simulink model "Sim_Forcing_003h_expe_infra5_practice1"  (Simulink 7.4)
settings: Solver=FixedStepDiscrete  StartTime=0.0  StopTime=inf  FixedStep=0.004  RelTol=1e-3
undefined symbols (not defined in the file or in its folder): DiscIntNeverNeededParam
libraries: simulink x24, gt_rt_lib x20, xpcutilitieslib x3, xpclib x2
(part 2 of 3)

== system Sim_Forcing_003h_expe_infra5_practice1/BEC (May 7, 2015)/CAN Receive/Convert 4*uni8 to int3 ==
  byte0 : Inport
  byte1 : Inport  Port=2
  byte2 : Inport  Port=3
  byte3 : Inport  Port=4
  Add : Sum  Inputs=++++  OutDataTypeMode=int32  OutDataType=fixdt(1, 16)  OutScaling=2^-10  OutDataTypeStr=int32
  Gain2 : Gain  Gain=256  ParameterDataType=fixdt(1, 16)  ParameterScaling=2^0  OutDataType=fixdt(1, 16)  OutScaling=2^0
  Gain3 : Gain  Gain=2^16  ParameterDataType=fixdt(1, 16)  ParameterScaling=2^0  OutDataType=fixdt(1, 16)  OutScaling=2^0
  Gain4 : Gain  Gain=2^24  ParameterDataType=fixdt(1, 16)  ParameterScaling=2^0  OutDataType=fixdt(1, 16)  OutScaling=2^0
  int : Outport
  wires:
  Gain4/1 -> Add/4
  byte3/1 -> Gain4/1
  byte2/1 -> Gain3/1
  byte1/1 -> Gain2/1
  Add/1 -> int/1
  byte0/1 -> Add/1
  Gain3/1 -> Add/3
  Gain2/1 -> Add/2

== system Sim_Forcing_003h_expe_infra5_practice1/BEC (May 7, 2015)/CAN Receive/Convert 4*uni8 to int4 ==
  byte0 : Inport
  byte1 : Inport  Port=2
  byte2 : Inport  Port=3
  byte3 : Inport  Port=4
  Add : Sum  Inputs=++++  OutDataTypeMode=int32  OutDataType=fixdt(1, 16)  OutScaling=2^-10  OutDataTypeStr=int32
  Gain2 : Gain  Gain=256  ParameterDataType=fixdt(1, 16)  ParameterScaling=2^0  OutDataType=fixdt(1, 16)  OutScaling=2^0
  Gain3 : Gain  Gain=2^16  ParameterDataType=fixdt(1, 16)  ParameterScaling=2^0  OutDataType=fixdt(1, 16)  OutScaling=2^0
  Gain4 : Gain  Gain=2^24  ParameterDataType=fixdt(1, 16)  ParameterScaling=2^0  OutDataType=fixdt(1, 16)  OutScaling=2^0
  int : Outport
  wires:
  Gain2/1 -> Add/2
  Gain3/1 -> Add/3
  byte0/1 -> Add/1
  Add/1 -> int/1
  byte1/1 -> Gain2/1
  byte2/1 -> Gain3/1
  byte3/1 -> Gain4/1
  Gain4/1 -> Add/4

== system Sim_Forcing_003h_expe_infra5_practice1/BEC (May 7, 2015)/CAN Receive/Convert 4*uni8 to int5 ==
  byte0 : Inport
  byte1 : Inport  Port=2
  byte2 : Inport  Port=3
  byte3 : Inport  Port=4
  Add : Sum  Inputs=++++  OutDataTypeMode=int32  OutDataType=fixdt(1, 16)  OutScaling=2^-10  OutDataTypeStr=int32
  Gain2 : Gain  Gain=256  ParameterDataType=fixdt(1, 16)  ParameterScaling=2^0  OutDataType=fixdt(1, 16)  OutScaling=2^0
  Gain3 : Gain  Gain=2^16  ParameterDataType=fixdt(1, 16)  ParameterScaling=2^0  OutDataType=fixdt(1, 16)  OutScaling=2^0
  Gain4 : Gain  Gain=2^24  ParameterDataType=fixdt(1, 16)  ParameterScaling=2^0  OutDataType=fixdt(1, 16)  OutScaling=2^0
  int : Outport
  wires:
  Gain4/1 -> Add/4
  byte3/1 -> Gain4/1
  byte2/1 -> Gain3/1
  byte1/1 -> Gain2/1
  Add/1 -> int/1
  byte0/1 -> Add/1
  Gain3/1 -> Add/3
  Gain2/1 -> Add/2

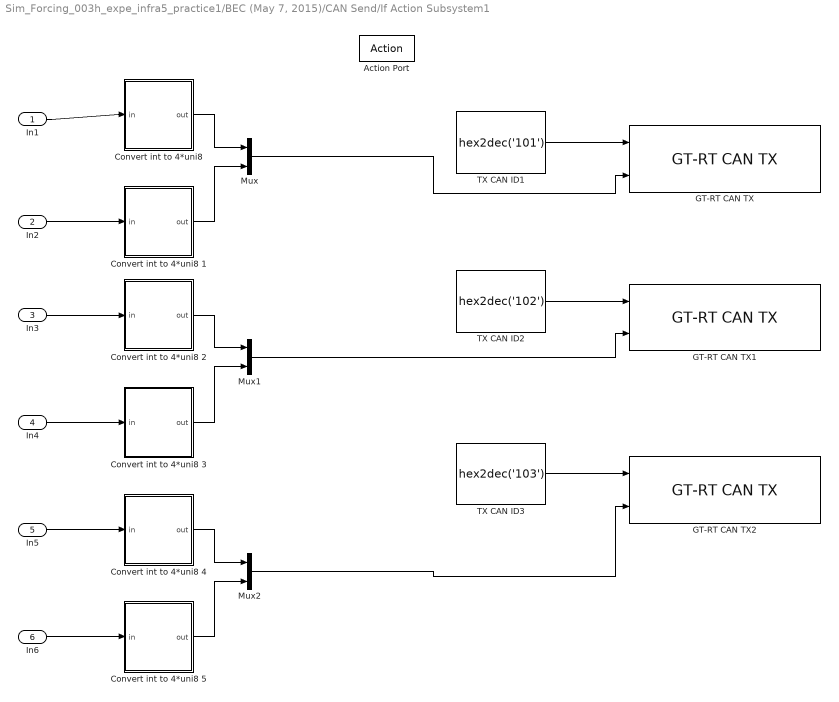
== system Sim_Forcing_003h_expe_infra5_practice1/BEC (May 7, 2015)/CAN Send/If Action Subsystem1 ==
  In1 : Inport  OutDataType=fixdt(1, 16)  OutScaling=2^0
  In2 : Inport  Port=2  OutDataType=fixdt(1, 16)  OutScaling=2^0
  In3 : Inport  Port=3  OutDataType=fixdt(1, 16)  OutScaling=2^0
  In4 : Inport  Port=4  OutDataType=fixdt(1, 16)  OutScaling=2^0
  In5 : Inport  Port=5  OutDataType=fixdt(1, 16)  OutScaling=2^0
  In6 : Inport  Port=6  OutDataType=fixdt(1, 16)  OutScaling=2^0
  Action Port : ActionPort  ActionType=then
  "Convert int to 4*uni8 " : Subsystem
  Convert int to 4*uni8 1 : Subsystem
  Convert int to 4*uni8 2 : Subsystem
  Convert int to 4*uni8 3 : Subsystem
  Convert int to 4*uni8 4 : Subsystem
  Convert int to 4*uni8 5 : Subsystem
  GT-RT CAN TX : gt_rt_lib/GT-RT CAN TX  uri='gt_rt_dev://localhost/dev/can0#0'  mff=MFF_11_DAT
  GT-RT CAN TX1 : gt_rt_lib/GT-RT CAN TX  uri='gt_rt_dev://localhost/dev/can0#0'  mff=MFF_11_DAT
  GT-RT CAN TX2 : gt_rt_lib/GT-RT CAN TX  uri='gt_rt_dev://localhost/dev/can0#0'  mff=MFF_11_DAT
  Mux : Mux  Inputs=2
  Mux1 : Mux  Inputs=2
  Mux2 : Mux  Inputs=2
  TX CAN ID1 : Constant  Value=hex2dec('101')  OutDataTypeMode=uint32  OutDataType=sfix(16)  OutScaling=2^0  OutDataTypeStr=uint32
  TX CAN ID2 : Constant  Value=hex2dec('102')  OutDataTypeMode=uint32  OutDataType=sfix(16)  OutScaling=2^0  OutDataTypeStr=uint32
  TX CAN ID3 : Constant  Value=hex2dec('103')  OutDataTypeMode=uint32  OutDataType=sfix(16)  OutScaling=2^0  OutDataTypeStr=uint32
  wires:
  In1/1 -> "Convert int to 4*uni8 "/1(in)
  In2/1 -> Convert int to 4*uni8 1/1(in)
  In3/1 -> Convert int to 4*uni8 2/1(in)
  In4/1 -> Convert int to 4*uni8 3/1(in)
  In5/1 -> Convert int to 4*uni8 4/1(in)
  In6/1 -> Convert int to 4*uni8 5/1(in)
  Mux2/1 -> GT-RT CAN TX2/2
  Convert int to 4*uni8 5/1(out) -> Mux2/2
  Convert int to 4*uni8 4/1(out) -> Mux2/1
  Mux1/1 -> GT-RT CAN TX1/2
  Convert int to 4*uni8 3/1(out) -> Mux1/2
  Convert int to 4*uni8 2/1(out) -> Mux1/1
  Mux/1 -> GT-RT CAN TX/2
  Convert int to 4*uni8 1/1(out) -> Mux/2
  "Convert int to 4*uni8 "/1(out) -> Mux/1
  TX CAN ID3/1 -> GT-RT CAN TX2/1
  TX CAN ID2/1 -> GT-RT CAN TX1/1
  TX CAN ID1/1 -> GT-RT CAN TX/1

== system Sim_Forcing_003h_expe_infra5_practice1/BEC (May 7, 2015)/Software limit switches/Subsystem ==
  In1 : Inport
  act : Inport  Port=2
  Abs1 : Abs  OutDataType=fixdt(1, 16)  OutScaling=2^0
  Abs2 : Abs  OutDataType=fixdt(1, 16)  OutScaling=2^0
  Add1 : Sum  Inputs=+-  OutDataType=fixdt(1, 16)  OutScaling=2^-10
  Add2 : Sum  Inputs=-+  OutDataType=fixdt(1, 16)  OutScaling=2^-10
  Display : Display
  Display2 : Display
  If Action Subsystem : Subsystem  TreatAsAtomicUnit=on
  If Action Subsystem1 : Subsystem  TreatAsAtomicUnit=on
  If2 : If
  NSEA1 : Constant  Value=-160  OutDataType=fixdt(1, 16)  OutScaling=2^0
  PSEA1 : Constant  Value=160  OutDataType=fixdt(1, 16)  OutScaling=2^0
  Switch : Switch  Criteria=u2 > Threshold  OutDataType=fixdt(1, 16)  OutScaling=2^0
  Switch1 : Switch  Criteria=u2 ~= 0  OutDataType=fixdt(1, 16)  OutScaling=2^0
  Out1 : Outport
  wires:
  If Action Subsystem1/1(Out1) -> Switch/3
  If Action Subsystem/1(Out1) -> Display/1, Switch/1
  Abs1/1 -> If Action Subsystem1/2(dif)
  If2/2 -> If Action Subsystem1/Action
  If2/1 -> If Action Subsystem/Action
  In1/1 -> If2/1, If Action Subsystem/2(Inc), If Action Subsystem1/1(Inc), Switch/2, Switch1/2, Switch1/3
  Abs2/1 -> If Action Subsystem/1(dif)
  NSEA1/1 -> Add1/2
  PSEA1/1 -> Add2/1
  Add1/1 -> Abs1/1
  Add2/1 -> Abs2/1
  Switch/1 -> Switch1/1
  Switch1/1 -> Out1/1, Display2/1
  act/1 -> Add1/1, Add2/2

== system Sim_Forcing_003h_expe_infra5_practice1/BEC (May 7, 2015)/Software limit switches/Subsystem1 ==
  In1 : Inport
  act : Inport  Port=2
  Abs1 : Abs  OutDataType=fixdt(1, 16)  OutScaling=2^0
  Abs2 : Abs  OutDataType=fixdt(1, 16)  OutScaling=2^0
  Add1 : Sum  Inputs=+-  OutDataType=fixdt(1, 16)  OutScaling=2^-10
  Add2 : Sum  Inputs=-+  OutDataType=fixdt(1, 16)  OutScaling=2^-10
  If Action Subsystem : Subsystem  TreatAsAtomicUnit=on
  If Action Subsystem1 : Subsystem  TreatAsAtomicUnit=on
  If2 : If
  NSEA1 : Constant  Value=-130  OutDataType=fixdt(1, 16)  OutScaling=2^0
  PSEA1 : Constant  Value=20  OutDataType=fixdt(1, 16)  OutScaling=2^0
  Switch : Switch  OutDataType=fixdt(1, 16)  OutScaling=2^0
  Switch1 : Switch  Criteria=u2 ~= 0  OutDataType=fixdt(1, 16)  OutScaling=2^0
  Out1 : Outport
  wires:
  act/1 -> Add1/1, Add2/2
  Add2/1 -> Abs2/1
  Add1/1 -> Abs1/1
  PSEA1/1 -> Add2/1
  NSEA1/1 -> Add1/2
  Abs2/1 -> If Action Subsystem/1(dif)
  In1/1 -> If Action Subsystem1/1(Inc), If Action Subsystem/2(Inc), Switch/2, Switch1/2, Switch1/3, If2/1
  If2/1 -> If Action Subsystem/Action
  If2/2 -> If Action Subsystem1/Action
  Abs1/1 -> If Action Subsystem1/2(dif)
  If Action Subsystem/1(Out1) -> Switch/1
  If Action Subsystem1/1(Out1) -> Switch/3
  Switch/1 -> Switch1/1
  Switch1/1 -> Out1/1

== system Sim_Forcing_003h_expe_infra5_practice1/BEC (May 7, 2015)/Software limit switches/Subsystem2 ==
  In1 : Inport
  act : Inport  Port=2
  Abs1 : Abs  OutDataType=fixdt(1, 16)  OutScaling=2^0
  Abs2 : Abs  OutDataType=fixdt(1, 16)  OutScaling=2^0
  Add1 : Sum  Inputs=+-  OutDataType=fixdt(1, 16)  OutScaling=2^-10
  Add2 : Sum  Inputs=-+  OutDataType=fixdt(1, 16)  OutScaling=2^-10
  If Action Subsystem : Subsystem  TreatAsAtomicUnit=on
  If Action Subsystem1 : Subsystem  TreatAsAtomicUnit=on
  If2 : If
  NSEA1 : Constant  Value=-88  OutDataType=fixdt(1, 16)  OutScaling=2^0
  PSEA1 : Constant  Value=88  OutDataType=fixdt(1, 16)  OutScaling=2^0
  Switch : Switch  OutDataType=fixdt(1, 16)  OutScaling=2^0
  Switch1 : Switch  Criteria=u2 ~= 0  OutDataType=fixdt(1, 16)  OutScaling=2^0
  Out1 : Outport
  wires:
  If Action Subsystem1/1(Out1) -> Switch/3
  If Action Subsystem/1(Out1) -> Switch/1
  Abs1/1 -> If Action Subsystem1/2(dif)
  If2/2 -> If Action Subsystem1/Action
  If2/1 -> If Action Subsystem/Action
  In1/1 -> If2/1, If Action Subsystem/2(Inc), If Action Subsystem1/1(Inc), Switch/2, Switch1/2, Switch1/3
  Abs2/1 -> If Action Subsystem/1(dif)
  NSEA1/1 -> Add1/2
  PSEA1/1 -> Add2/1
  Add1/1 -> Abs1/1
  Add2/1 -> Abs2/1
  act/1 -> Add1/1, Add2/2
  Switch/1 -> Switch1/1
  Switch1/1 -> Out1/1

== system Sim_Forcing_003h_expe_infra5_practice1/BEC (May 7, 2015)/Software limit switches/Subsystem3 ==
  In1 : Inport
  act : Inport  Port=2
  Abs1 : Abs  OutDataType=fixdt(1, 16)  OutScaling=2^0
  Abs2 : Abs  OutDataType=fixdt(1, 16)  OutScaling=2^0
  Add1 : Sum  Inputs=+-  OutDataType=fixdt(1, 16)  OutScaling=2^-10
  Add2 : Sum  Inputs=-+  OutDataType=fixdt(1, 16)  OutScaling=2^-10
  If Action Subsystem : Subsystem  TreatAsAtomicUnit=on
  If Action Subsystem1 : Subsystem  TreatAsAtomicUnit=on
  If2 : If
  NSEA1 : Constant  Value=-350  OutDataType=fixdt(1, 16)  OutScaling=2^0
  PSEA1 : Constant  Value=350  OutDataType=fixdt(1, 16)  OutScaling=2^0
  Switch : Switch  OutDataType=fixdt(1, 16)  OutScaling=2^0
  Switch1 : Switch  Criteria=u2 ~= 0  OutDataType=fixdt(1, 16)  OutScaling=2^0
  Out1 : Outport
  wires:
  Add2/1 -> Abs2/1
  Add1/1 -> Abs1/1
  PSEA1/1 -> Add2/1
  NSEA1/1 -> Add1/2
  Abs2/1 -> If Action Subsystem/1(dif)
  In1/1 -> If Action Subsystem1/1(Inc), If Action Subsystem/2(Inc), Switch/2, Switch1/2, Switch1/3, If2/1
  If2/1 -> If Action Subsystem/Action
  If2/2 -> If Action Subsystem1/Action
  act/1 -> Add2/2, Add1/1
  Abs1/1 -> If Action Subsystem1/2(dif)
  If Action Subsystem/1(Out1) -> Switch/1
  If Action Subsystem1/1(Out1) -> Switch/3
  Switch/1 -> Switch1/1
  Switch1/1 -> Out1/1

== system Sim_Forcing_003h_expe_infra5_practice1/BEC (May 7, 2015)/Software limit switches/Subsystem4 ==
  In1 : Inport
  act : Inport  Port=2
  Abs1 : Abs  OutDataType=fixdt(1, 16)  OutScaling=2^0
  Abs2 : Abs  OutDataType=fixdt(1, 16)  OutScaling=2^0
  Add1 : Sum  Inputs=+-  OutDataType=fixdt(1, 16)  OutScaling=2^-10
  Add2 : Sum  Inputs=-+  OutDataType=fixdt(1, 16)  OutScaling=2^-10
  If Action Subsystem : Subsystem  TreatAsAtomicUnit=on
  If Action Subsystem1 : Subsystem  TreatAsAtomicUnit=on
  If2 : If
  NSEA1 : Constant  Value=-61  OutDataType=fixdt(1, 16)  OutScaling=2^0
  PSEA1 : Constant  Value=61  OutDataType=fixdt(1, 16)  OutScaling=2^0
  Switch : Switch  OutDataType=fixdt(1, 16)  OutScaling=2^0
  Switch1 : Switch  Criteria=u2 ~= 0  OutDataType=fixdt(1, 16)  OutScaling=2^0
  Out1 : Outport
  wires:
  If Action Subsystem/1(Out1) -> Switch/1
  Abs1/1 -> If Action Subsystem1/2(dif)
  If2/2 -> If Action Subsystem1/Action
  If2/1 -> If Action Subsystem/Action
  In1/1 -> If2/1, If Action Subsystem/2(Inc), If Action Subsystem1/1(Inc), Switch/2, Switch1/2, Switch1/3
  Abs2/1 -> If Action Subsystem/1(dif)
  NSEA1/1 -> Add1/2
  PSEA1/1 -> Add2/1
  Add1/1 -> Abs1/1
  Add2/1 -> Abs2/1
  If Action Subsystem1/1(Out1) -> Switch/3
  Switch/1 -> Switch1/1
  Switch1/1 -> Out1/1
  act/1 -> Add2/2, Add1/1

== system Sim_Forcing_003h_expe_infra5_practice1/BEC (May 7, 2015)/Software limit switches/Subsystem5 ==
  In1 : Inport
  act : Inport  Port=2
  Abs1 : Abs  OutDataType=fixdt(1, 16)  OutScaling=2^0
  Abs2 : Abs  OutDataType=fixdt(1, 16)  OutScaling=2^0
  Add1 : Sum  Inputs=+-  OutDataType=fixdt(1, 16)  OutScaling=2^-10
  Add2 : Sum  Inputs=-+  OutDataType=fixdt(1, 16)  OutScaling=2^-10
  If Action Subsystem : Subsystem  TreatAsAtomicUnit=on
  If Action Subsystem1 : Subsystem  TreatAsAtomicUnit=on
  If2 : If
  NSEA1 : Constant  Value=-350  OutDataType=fixdt(1, 16)  OutScaling=2^0
  PSEA1 : Constant  Value=350  OutDataType=fixdt(1, 16)  OutScaling=2^0
  Switch : Switch  OutDataType=fixdt(1, 16)  OutScaling=2^0
  Switch1 : Switch  Criteria=u2 ~= 0  OutDataType=fixdt(1, 16)  OutScaling=2^0
  Out1 : Outport
  wires:
  Add2/1 -> Abs2/1
  Add1/1 -> Abs1/1
  PSEA1/1 -> Add2/1
  NSEA1/1 -> Add1/2
  Abs2/1 -> If Action Subsystem/1(dif)
  In1/1 -> If Action Subsystem1/1(Inc), If Action Subsystem/2(Inc), Switch/2, Switch1/2, Switch1/3, If2/1
  If2/1 -> If Action Subsystem/Action
  If2/2 -> If Action Subsystem1/Action
  Abs1/1 -> If Action Subsystem1/2(dif)
  If Action Subsystem/1(Out1) -> Switch/1
  If Action Subsystem1/1(Out1) -> Switch/3
  Switch/1 -> Switch1/1
  Switch1/1 -> Out1/1
  act/1 -> Add2/2, Add1/1

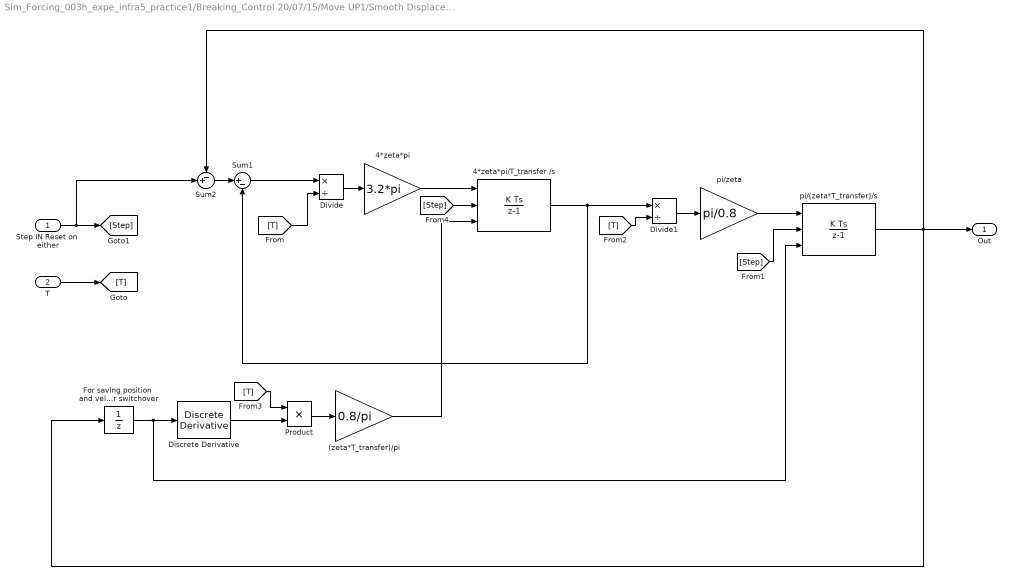
== system Sim_Forcing_003h_expe_infra5_practice1/Breaking_Control 20/07/15/Move UP1/Smooth Displacement Second-Order Filter, zeta 0.8 ==
  Step IN Reset on  either : Inport
  T : Inport  Port=2  OutDataType=fixdt(1, 16)  OutScaling=2^0
  (zeta*T_transfer)/pi : Gain  Gain=0.8/pi  ParameterDataType=fixdt(1, 16)  ParameterScaling=2^0  OutDataType=fixdt(1, 16)  OutScaling=2^0
  4*zeta*pi : Gain  Gain=3.2*pi  ParameterDataType=fixdt(1, 16)  ParameterScaling=2^0  OutDataType=fixdt(1, 16)  OutScaling=2^0
  4*zeta*pi/T_transfer /s : DiscreteIntegrator  gainval=1  ExternalReset=either  InitialConditionSource=external  SampleTime=0.004  OutDataType=fixdt(1, 16)  OutScaling=2^0  ICPrevOutput=DiscIntNeverNeededParam  ICPrevScaledInput=DiscIntNeverNeededParam
  Discrete Derivative : simulink/Discrete/Discrete Derivative  SystemSampleTime=-1  gainval=1.0  ICPrevScaledInput=0.0  OutMin=[]  OutMax=[]  OutDataType=fixdt(1, 16)  OutScaling=2^-10  DoSatur=off
  Divide : Product  Inputs=*/  OutDataType=fixdt(1, 16)  OutScaling=2^-10
  Divide1 : Product  Inputs=*/  OutDataType=fixdt(1, 16)  OutScaling=2^-10
  For saving position  and velocity until after switchover : UnitDelay  SampleTime=-1
  Product : Product  OutDataType=fixdt(1, 16)  OutScaling=2^0  RndMeth=Zero
  Sum1 : Sum  Inputs=|+-  OutDataType=fixdt(1, 16)  OutScaling=2^0
  Sum2 : Sum  Inputs=-+|  OutDataType=fixdt(1, 16)  OutScaling=2^0
  pi/(zeta*T_transfer)/s : DiscreteIntegrator  gainval=1  ExternalReset=either  InitialConditionSource=external  SampleTime=0.004  OutDataType=fixdt(1, 16)  OutScaling=2^0  ICPrevOutput=DiscIntNeverNeededParam  ICPrevScaledInput=DiscIntNeverNeededParam
  pi/zeta : Gain  Gain=pi/0.8  ParameterDataType=fixdt(1, 16)  ParameterScaling=2^0  OutDataType=fixdt(1, 16)  OutScaling=2^0
  Out : Outport
  wires:
  Discrete Derivative/1 -> Product/2
  Product/1 -> (zeta*T_transfer)/pi/1
  Divide/1 -> 4*zeta*pi/1
  Divide1/1 -> pi/zeta/1
  pi/zeta/1 -> pi/(zeta*T_transfer)/s/1
  pi/(zeta*T_transfer)/s/1 -> Sum2/1, Out/1, For saving position  and velocity until after switchover/1
  4*zeta*pi/T_transfer /s/1 -> Divide1/1, Sum1/2
  Sum1/1 -> Divide/1
  4*zeta*pi/1 -> 4*zeta*pi/T_transfer /s/1
  T/1 -> [T]
  Step IN Reset on  either/1 -> [Step], Sum2/2
  [Step] -> 4*zeta*pi/T_transfer /s/2
  [Step] -> pi/(zeta*T_transfer)/s/2
  [T] -> Divide/2
  For saving position  and velocity until after switchover/1 -> Discrete Derivative/1, pi/(zeta*T_transfer)/s/3
  [T] -> Product/1
  (zeta*T_transfer)/pi/1 -> 4*zeta*pi/T_transfer /s/3
  [T] -> Divide1/2
  Sum2/1 -> Sum1/1

== system Sim_Forcing_003h_expe_infra5_practice1/Breaking_Control 20/07/15/Move UP1/add x_offset ==
  x_offset : Inport
  set_in : Inport  Port=2
  Embedded MATLAB Function : Stateflow chart
  set_out : Outport
  wires:
  x_offset/1 -> Embedded MATLAB Function/1(dx)
  Embedded MATLAB Function/1(set_out) -> set_out/1
  set_in/1 -> Embedded MATLAB Function/2(set_in)

== system Sim_Forcing_003h_expe_infra5_practice1/Breaking_Control 20/07/15/practice_phase1/Rate Control Dynamics Phi ==
  Turn_rate_roll (deg/sec) : Inport
  practice : Inport  Port=2
  reset from_connect_y : Inport  Port=3
  Constant : Constant  Value=0.1  OutDataType=fixdt(1, 16)  OutScaling=2^0
  Constant1 : Constant  Value=15  OutDataType=fixdt(1, 16)  OutScaling=2^0
  Constant3 : Constant  Value=0.1  OutDataType=fixdt(1, 16)  OutScaling=2^0
  Discrete-Time Integrator1 : DiscreteIntegrator  ExternalReset=either  SampleTime=0.004  OutDataType=fixdt(1, 16)  OutScaling=2^0  ICPrevOutput=DiscIntNeverNeededParam  ICPrevScaledInput=DiscIntNeverNeededParam
  Limit to 5 : Saturate  UpperLimit=5  LowerLimit=-5  OutDataType=fixdt(1, 16)  OutScaling=2^0
  Product : Product  OutDataType=fixdt(1, 16)  OutScaling=2^0  RndMeth=Zero
  "Second-Order Filter, zeta 0.8" : Subsystem
  "Smooth Displacement Second-Order Filter, zeta 0.8" : Subsystem
  Switch : Switch  Criteria=u2 > Threshold  OutDataType=fixdt(1, 16)  OutScaling=2^0
  phi (deg) : Outport
  wires:
  Turn_rate_roll (deg/sec)/1 -> "Second-Order Filter, zeta 0.8"/1(u)
  "Second-Order Filter, zeta 0.8"/1(x) -> Limit to 5/1
  Constant/1 -> "Second-Order Filter, zeta 0.8"/2(T)
  Discrete-Time Integrator1/1 -> Product/1
  Product/1 -> phi (deg)/1
  "Smooth Displacement Second-Order Filter, zeta 0.8"/1(Out) -> Product/2
  Limit to 5/1 -> Discrete-Time Integrator1/1
  practice/1 -> "Smooth Displacement Second-Order Filter, zeta 0.8"/1(Step IN Reset on  either), Switch/2
  reset from_connect_y/1 -> Discrete-Time Integrator1/2
  Constant3/1 -> Switch/1
  Constant1/1 -> Switch/3
  Switch/1 -> "Smooth Displacement Second-Order Filter, zeta 0.8"/2(T)

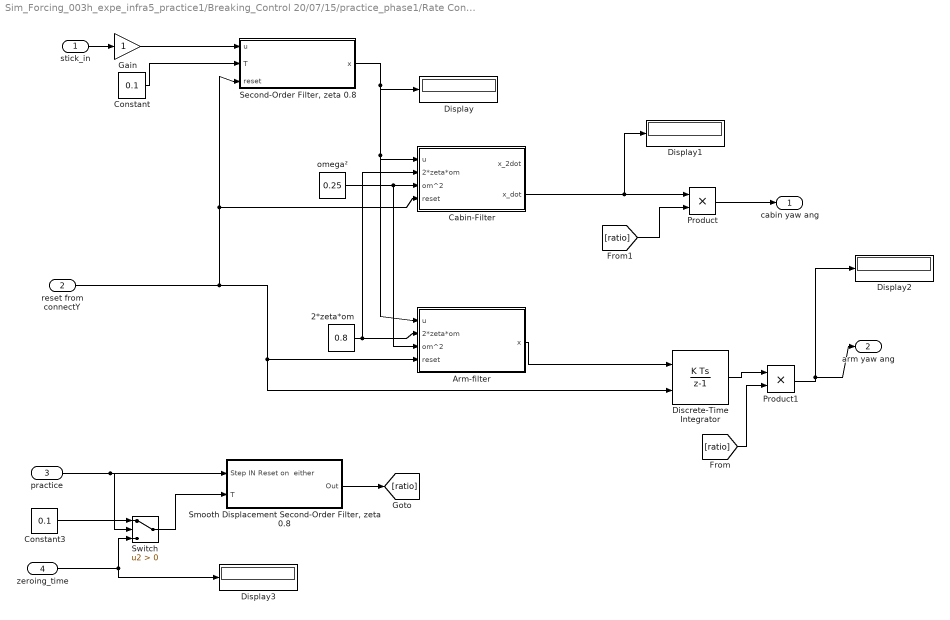
== system Sim_Forcing_003h_expe_infra5_practice1/Breaking_Control 20/07/15/practice_phase1/Rate Control Dynamics Psi2 ==
  stick_in : Inport  OutDataType=fixdt(1, 16)  OutScaling=2^0
  reset from connectY : Inport  Port=2  OutDataType=fixdt(1, 16)  OutScaling=2^0
  practice : Inport  Port=3
  zeroing_time : Inport  Port=4
  2*zeta*om : Constant  Value=0.8
  Arm-filter : Subsystem
  Cabin-Filter : Subsystem
  Constant : Constant  Value=0.1  OutDataType=fixdt(1, 16)  OutScaling=2^0
  Constant3 : Constant  Value=0.1  OutDataType=fixdt(1, 16)  OutScaling=2^0
  Discrete-Time Integrator : DiscreteIntegrator  ExternalReset=either  SampleTime=0.004  ICPrevOutput=DiscIntNeverNeededParam  ICPrevScaledInput=DiscIntNeverNeededParam
  Display{,1..3} (4 alike) : Display
  Gain : Gain  ParameterDataType=fixdt(1, 16)  ParameterScaling=2^0  OutDataType=fixdt(1, 16)  OutScaling=2^0
  Product : Product  OutDataType=fixdt(1, 16)  OutScaling=2^0  RndMeth=Zero
  Product1 : Product  OutDataType=fixdt(1, 16)  OutScaling=2^0  RndMeth=Zero
  "Second-Order Filter, zeta 0.8" : Subsystem
  "Smooth Displacement Second-Order Filter, zeta 0.8" : Subsystem
  Switch : Switch  Criteria=u2 > Threshold  OutDataType=fixdt(1, 16)  OutScaling=2^0
  omega² : Constant  Value=0.25
  cabin yaw ang : Outport  OutDataType=fixdt(1, 16)  OutScaling=2^0
  arm yaw ang : Outport  Port=2  OutDataType=fixdt(1, 16)  OutScaling=2^0
  wires:
  Arm-filter/1(x) -> Discrete-Time Integrator/1
  stick_in/1 -> Gain/1
  omega²/1 -> Arm-filter/3(om^2), Cabin-Filter/3(om^2)
  2*zeta*om/1 -> Arm-filter/2(2*zeta*om), Cabin-Filter/2(2*zeta*om)
  Cabin-Filter/2(x_dot) -> Display1/1, Product/1
  reset from connectY/1 -> Cabin-Filter/4(reset), "Second-Order Filter, zeta 0.8"/3(reset), Arm-filter/4(reset), Discrete-Time Integrator/2
  Constant/1 -> "Second-Order Filter, zeta 0.8"/2(T)
  "Second-Order Filter, zeta 0.8"/1(x) -> Cabin-Filter/1(u), Arm-filter/1(u), Display/1
  Gain/1 -> "Second-Order Filter, zeta 0.8"/1(u)
  Constant3/1 -> Switch/1
  zeroing_time/1 -> Switch/3, Display3/1
  Switch/1 -> "Smooth Displacement Second-Order Filter, zeta 0.8"/2(T)
  practice/1 -> Switch/2, "Smooth Displacement Second-Order Filter, zeta 0.8"/1(Step IN Reset on  either)
  "Smooth Displacement Second-Order Filter, zeta 0.8"/1(Out) -> [ratio]
  Product/1 -> cabin yaw ang/1
  Discrete-Time Integrator/1 -> Product1/1
  Product1/1 -> Display2/1, arm yaw ang/1
  [ratio] -> Product1/2
  [ratio] -> Product/2

== system Sim_Forcing_003h_expe_infra5_practice1/Breaking_Control 20/07/15/practice_phase1/Rate Control Dynamics Theta ==
  Turn_rate_pitch (deg/sec) : Inport
  practice : Inport  Port=2
  reset from_connect_y : Inport  Port=3
  Constant : Constant  Value=0.1  OutDataType=fixdt(1, 16)  OutScaling=2^0
  Constant1 : Constant  Value=15  OutDataType=fixdt(1, 16)  OutScaling=2^0
  Constant2 : Constant  Value=0.1  OutDataType=fixdt(1, 16)  OutScaling=2^0
  Discrete-Time Integrator1 : DiscreteIntegrator  ExternalReset=either  SampleTime=0.004  OutDataType=fixdt(1, 16)  OutScaling=2^0  ICPrevOutput=DiscIntNeverNeededParam  ICPrevScaledInput=DiscIntNeverNeededParam
  Limit to 5 : Saturate  UpperLimit=5  LowerLimit=-5  OutDataType=fixdt(1, 16)  OutScaling=2^0
  Product : Product  OutDataType=fixdt(1, 16)  OutScaling=2^0  RndMeth=Zero
  "Second-Order Filter, zeta 0.8" : Subsystem
  "Smooth Displacement Second-Order Filter, zeta 0.8" : Subsystem
  Switch : Switch  Criteria=u2 > Threshold  OutDataType=fixdt(1, 16)  OutScaling=2^0
  theta (deg) : Outport
  wires:
  Turn_rate_pitch (deg/sec)/1 -> "Second-Order Filter, zeta 0.8"/1(u)
  "Second-Order Filter, zeta 0.8"/1(x) -> Limit to 5/1
  Constant/1 -> "Second-Order Filter, zeta 0.8"/2(T)
  Discrete-Time Integrator1/1 -> Product/1
  Product/1 -> theta (deg)/1
  "Smooth Displacement Second-Order Filter, zeta 0.8"/1(Out) -> Product/2
  Limit to 5/1 -> Discrete-Time Integrator1/1
  reset from_connect_y/1 -> Discrete-Time Integrator1/2
  practice/1 -> "Smooth Displacement Second-Order Filter, zeta 0.8"/1(Step IN Reset on  either), Switch/2
  Switch/1 -> "Smooth Displacement Second-Order Filter, zeta 0.8"/2(T)
  Constant2/1 -> Switch/1
  Constant1/1 -> Switch/3

== system Sim_Forcing_003h_expe_infra5_practice1/Joint Controller (May 7, 2015)1/Forward Kinematics/KUKA2NED ==
  KUKA : Inport
  Constant : Constant  Value=[0 0 0 0 0 15.89]  OutDataType=fixdt(1, 16)  OutScaling=2^0
  Gain : Gain  Gain=[1 -1 -1 -1 -1 -1]  ParameterDataType=fixdt(1, 16)  ParameterScaling=2^0  OutDataType=fixdt(1, 16)  OutScaling=2^0
  Sum : Sum  Inputs=|++  OutDataType=fixdt(1, 16)  OutScaling=2^0
  NED : Outport
  wires:
  Gain/1 -> Sum/1
  KUKA/1 -> Gain/1
  Sum/1 -> NED/1
  Constant/1 -> Sum/2

== system Sim_Forcing_003h_expe_infra5_practice1/Joint Controller (May 7, 2015)1/Inverse Kinematics May 6, 2015/Inverse Kinematics ==
  note: (6_DOF_ACT - 6_DOF_COM) exp(-0.1t) + 6_DOF_COM
  vec : Inport
  Activate full inverse : Inport  Port=2
  6_DOF_ACT : Inport  Port=3  OutDataType=fixdt(1, 16)  OutScaling=2^0
  Demux : Demux  Outputs=[6,6]
  Discrete-Time Integrator : DiscreteIntegrator  gainval=1  ExternalReset=either  InitialConditionSource=external  SampleTime=-1  OutDataType=fixdt(1, 16)  OutScaling=2^0  ICPrevOutput=DiscIntNeverNeededParam  ICPrevScaledInput=DiscIntNeverNeededParam
  Gain : Gain  Gain=-0.1  ParameterDataType=fixdt(1, 16)  ParameterScaling=2^0  OutDataType=fixdt(1, 16)  OutScaling=2^0
  Mux : Mux  Inputs=2
  Select -6_DOF_COM : Selector  InputPortWidth=12  IndexOptions=Index vector (dialog)  Indices=[1 2 3 4 5 6]  OutputSizes=1
  Sum : Sum  Inputs=|-+  OutDataType=fixdt(1, 16)  OutScaling=2^0
  Sum1 : Sum  Inputs=|++  OutDataType=fixdt(1, 16)  OutScaling=2^0
  full inverse kin : Subsystem
  out : Outport  OutDataType=fixdt(1, 16)  OutScaling=2^0
  wires:
  vec/1 -> Select -6_DOF_COM/1, Demux/1
  full inverse kin/1(out) -> out/1
  Activate full inverse/1 -> full inverse kin/Enable, Discrete-Time Integrator/2
  Discrete-Time Integrator/1 -> Gain/1, Sum1/2
  Gain/1 -> Discrete-Time Integrator/1
  6_DOF_ACT/1 -> Sum/2
  Select -6_DOF_COM/1 -> Sum/1
  Sum/1 -> Discrete-Time Integrator/3
  Demux/2 -> Mux/2
  Demux/1 -> Sum1/1
  Sum1/1 -> Mux/1
  Mux/1 -> full inverse kin/1(vec)

== system Sim_Forcing_003h_expe_infra5_practice1/Joint Controller (May 7, 2015)1/Inverse Kinematics May 6, 2015/NED2KUKA ==
  NED : Inport
  Constant : Constant  Value=[0 0 0 0 0 15.89]  OutDataType=fixdt(1, 16)  OutScaling=2^0
  Gain : Gain  Gain=[1 -1 -1 -1 -1 -1]  ParameterDataType=fixdt(1, 16)  ParameterScaling=2^0  OutDataType=fixdt(1, 16)  OutScaling=2^0
  Sum : Sum  Inputs=|++  OutDataType=fixdt(1, 16)  OutScaling=2^0
  KUKA : Outport
  wires:
  Gain/1 -> Sum/1
  NED/1 -> Gain/1
  Sum/1 -> KUKA/1
  Constant/1 -> Sum/2

== system Sim_Forcing_003h_expe_infra5_practice1/Joint Controller (May 7, 2015)1/Inverse Kinematics May 6, 2015/Simplified Inverse Kinematics ==
  note: (A1-A6_ACT - A1-A6_COM) exp(-0.1t) + A1-A6_COM
  note: Selects and sets
      |  A1, A4,A6 to zero
  note: This version has been tested on May 6, 2015
  activate simplified : Inport  OutDataType=fixdt(1, 16)  OutScaling=2^0
  vec : Inport  Port=2  OutDataType=fixdt(1, 16)  OutScaling=2^0
  A1-A6 ACT : Selector  InputPortWidth=12  IndexOptions=Index vector (dialog)  Indices=[7 8 9 10 11 12]  OutputSizes=1
  A1-A6 COM : Subsystem
  Discrete-Time Integrator1 : DiscreteIntegrator  gainval=1  ExternalReset=either  InitialConditionSource=external  SampleTime=-1  OutDataType=fixdt(1, 16)  OutScaling=2^0  ICPrevOutput=DiscIntNeverNeededParam  ICPrevScaledInput=DiscIntNeverNeededParam
  Gain1 : Gain  Gain=-0.1  ParameterDataType=fixdt(1, 16)  ParameterScaling=2^0  OutDataType=fixdt(1, 16)  OutScaling=2^0
  Mux : Mux  Inputs=2
  N : Selector  InputPortWidth=7  IndexOptions=Index vector (dialog)  Indices=7  OutputSizes=1
  Simplified Inverse Kin : Subsystem
  Sum : Sum  Inputs=-+|  OutDataType=fixdt(1, 16)  OutScaling=2^0
  Sum1 : Sum  Inputs=++|  OutDataType=fixdt(1, 16)  OutScaling=2^0
  out : Outport  OutDataType=fixdt(1, 16)  OutScaling=2^0
  wires:
  vec/1 -> Simplified Inverse Kin/1(Vec), A1-A6 ACT/1
  activate simplified/1 -> Simplified Inverse Kin/Enable, Discrete-Time Integrator1/2
  Discrete-Time Integrator1/1 -> Gain1/1, Sum1/2
  Gain1/1 -> Discrete-Time Integrator1/1
  Sum1/1 -> Mux/1
  Sum/1 -> Discrete-Time Integrator1/3
  Mux/1 -> out/1
  A1-A6 ACT/1 -> Sum/2
  Simplified Inverse Kin/1(Out) -> A1-A6 COM/1(vec), N/1
  A1-A6 COM/1(A1-A6 COM) -> Sum/1, Sum1/1
  N/1 -> Mux/2

== system Sim_Forcing_003h_expe_infra5_practice1/BEC (May 7, 2015)/CAN Send/If Action Subsystem1/Convert int to 4*uni8  ==
  in : Inport
  Gain{1..4} (4 alike) : Gain  ParameterDataType=fixdt(1, 16)  ParameterScaling=2^0  OutDataTypeMode=uint8  OutDataType=fixdt(1, 16)  OutScaling=2^0  OutDataTypeStr=uint8
  Mux : Mux
  Shift Arithmetic : simulink/Logic and Bit Operations/Shift Arithmetic  SystemSampleTime=-1  nBitShiftRight=8  nBinPtShiftRight=0
  Shift Arithmetic1 : simulink/Logic and Bit Operations/Shift Arithmetic  SystemSampleTime=-1  nBitShiftRight=16  nBinPtShiftRight=0
  Shift Arithmetic2 : simulink/Logic and Bit Operations/Shift Arithmetic  SystemSampleTime=-1  nBitShiftRight=24  nBinPtShiftRight=0
  out : Outport
  wires:
  in/1 -> Shift Arithmetic1/1, Gain1/1, Shift Arithmetic/1, Shift Arithmetic2/1
  Shift Arithmetic/1 -> Gain2/1
  Shift Arithmetic1/1 -> Gain3/1
  Shift Arithmetic2/1 -> Gain4/1
  Gain1/1 -> Mux/1
  Gain2/1 -> Mux/2
  Gain3/1 -> Mux/3
  Gain4/1 -> Mux/4
  Mux/1 -> out/1

== system Sim_Forcing_003h_expe_infra5_practice1/BEC (May 7, 2015)/CAN Send/If Action Subsystem1/Convert int to 4*uni8 1 ==
  in : Inport
  Gain{1..4} (4 alike) : Gain  ParameterDataType=fixdt(1, 16)  ParameterScaling=2^0  OutDataTypeMode=uint8  OutDataType=fixdt(1, 16)  OutScaling=2^0  OutDataTypeStr=uint8
  Mux : Mux
  Shift Arithmetic : simulink/Logic and Bit Operations/Shift Arithmetic  SystemSampleTime=-1  nBitShiftRight=8  nBinPtShiftRight=0
  Shift Arithmetic1 : simulink/Logic and Bit Operations/Shift Arithmetic  SystemSampleTime=-1  nBitShiftRight=16  nBinPtShiftRight=0
  Shift Arithmetic2 : simulink/Logic and Bit Operations/Shift Arithmetic  SystemSampleTime=-1  nBitShiftRight=24  nBinPtShiftRight=0
  out : Outport
  wires:
  Mux/1 -> out/1
  Gain4/1 -> Mux/4
  Gain3/1 -> Mux/3
  Gain2/1 -> Mux/2
  Gain1/1 -> Mux/1
  Shift Arithmetic2/1 -> Gain4/1
  Shift Arithmetic1/1 -> Gain3/1
  Shift Arithmetic/1 -> Gain2/1
  in/1 -> Shift Arithmetic2/1, Shift Arithmetic/1, Gain1/1, Shift Arithmetic1/1

== system Sim_Forcing_003h_expe_infra5_practice1/BEC (May 7, 2015)/CAN Send/If Action Subsystem1/Convert int to 4*uni8 2 ==
  in : Inport
  Gain{1..4} (4 alike) : Gain  ParameterDataType=fixdt(1, 16)  ParameterScaling=2^0  OutDataTypeMode=uint8  OutDataType=fixdt(1, 16)  OutScaling=2^0  OutDataTypeStr=uint8
  Mux : Mux
  Shift Arithmetic : simulink/Logic and Bit Operations/Shift Arithmetic  SystemSampleTime=-1  nBitShiftRight=8  nBinPtShiftRight=0
  Shift Arithmetic1 : simulink/Logic and Bit Operations/Shift Arithmetic  SystemSampleTime=-1  nBitShiftRight=16  nBinPtShiftRight=0
  Shift Arithmetic2 : simulink/Logic and Bit Operations/Shift Arithmetic  SystemSampleTime=-1  nBitShiftRight=24  nBinPtShiftRight=0
  out : Outport
  wires:
  Mux/1 -> out/1
  Gain4/1 -> Mux/4
  Gain3/1 -> Mux/3
  Gain2/1 -> Mux/2
  Gain1/1 -> Mux/1
  Shift Arithmetic2/1 -> Gain4/1
  Shift Arithmetic1/1 -> Gain3/1
  Shift Arithmetic/1 -> Gain2/1
  in/1 -> Shift Arithmetic2/1, Shift Arithmetic/1, Gain1/1, Shift Arithmetic1/1

== system Sim_Forcing_003h_expe_infra5_practice1/BEC (May 7, 2015)/CAN Send/If Action Subsystem1/Convert int to 4*uni8 3 ==
  in : Inport
  Gain{1..4} (4 alike) : Gain  ParameterDataType=fixdt(1, 16)  ParameterScaling=2^0  OutDataTypeMode=uint8  OutDataType=fixdt(1, 16)  OutScaling=2^0  OutDataTypeStr=uint8
  Mux : Mux
  Shift Arithmetic : simulink/Logic and Bit Operations/Shift Arithmetic  SystemSampleTime=-1  nBitShiftRight=8  nBinPtShiftRight=0
  Shift Arithmetic1 : simulink/Logic and Bit Operations/Shift Arithmetic  SystemSampleTime=-1  nBitShiftRight=16  nBinPtShiftRight=0
  Shift Arithmetic2 : simulink/Logic and Bit Operations/Shift Arithmetic  SystemSampleTime=-1  nBitShiftRight=24  nBinPtShiftRight=0
  out : Outport
  wires:
  in/1 -> Shift Arithmetic1/1, Gain1/1, Shift Arithmetic/1, Shift Arithmetic2/1
  Shift Arithmetic/1 -> Gain2/1
  Shift Arithmetic1/1 -> Gain3/1
  Shift Arithmetic2/1 -> Gain4/1
  Gain1/1 -> Mux/1
  Gain2/1 -> Mux/2
  Gain3/1 -> Mux/3
  Gain4/1 -> Mux/4
  Mux/1 -> out/1

== system Sim_Forcing_003h_expe_infra5_practice1/BEC (May 7, 2015)/CAN Send/If Action Subsystem1/Convert int to 4*uni8 4 ==
  in : Inport
  Gain{1..4} (4 alike) : Gain  ParameterDataType=fixdt(1, 16)  ParameterScaling=2^0  OutDataTypeMode=uint8  OutDataType=fixdt(1, 16)  OutScaling=2^0  OutDataTypeStr=uint8
  Mux : Mux
  Shift Arithmetic : simulink/Logic and Bit Operations/Shift Arithmetic  SystemSampleTime=-1  nBitShiftRight=8  nBinPtShiftRight=0
  Shift Arithmetic1 : simulink/Logic and Bit Operations/Shift Arithmetic  SystemSampleTime=-1  nBitShiftRight=16  nBinPtShiftRight=0
  Shift Arithmetic2 : simulink/Logic and Bit Operations/Shift Arithmetic  SystemSampleTime=-1  nBitShiftRight=24  nBinPtShiftRight=0
  out : Outport
  wires:
  in/1 -> Shift Arithmetic1/1, Gain1/1, Shift Arithmetic/1, Shift Arithmetic2/1
  Shift Arithmetic/1 -> Gain2/1
  Shift Arithmetic1/1 -> Gain3/1
  Shift Arithmetic2/1 -> Gain4/1
  Gain1/1 -> Mux/1
  Gain2/1 -> Mux/2
  Gain3/1 -> Mux/3
  Gain4/1 -> Mux/4
  Mux/1 -> out/1

== system Sim_Forcing_003h_expe_infra5_practice1/BEC (May 7, 2015)/CAN Send/If Action Subsystem1/Convert int to 4*uni8 5 ==
  in : Inport
  Gain{1..4} (4 alike) : Gain  ParameterDataType=fixdt(1, 16)  ParameterScaling=2^0  OutDataTypeMode=uint8  OutDataType=fixdt(1, 16)  OutScaling=2^0  OutDataTypeStr=uint8
  Mux : Mux
  Shift Arithmetic : simulink/Logic and Bit Operations/Shift Arithmetic  SystemSampleTime=-1  nBitShiftRight=8  nBinPtShiftRight=0
  Shift Arithmetic1 : simulink/Logic and Bit Operations/Shift Arithmetic  SystemSampleTime=-1  nBitShiftRight=16  nBinPtShiftRight=0
  Shift Arithmetic2 : simulink/Logic and Bit Operations/Shift Arithmetic  SystemSampleTime=-1  nBitShiftRight=24  nBinPtShiftRight=0
  out : Outport
  wires:
  Mux/1 -> out/1
  Gain4/1 -> Mux/4
  Gain3/1 -> Mux/3
  Gain2/1 -> Mux/2
  Gain1/1 -> Mux/1
  Shift Arithmetic2/1 -> Gain4/1
  Shift Arithmetic1/1 -> Gain3/1
  Shift Arithmetic/1 -> Gain2/1
  in/1 -> Shift Arithmetic2/1, Shift Arithmetic/1, Gain1/1, Shift Arithmetic1/1

== system Sim_Forcing_003h_expe_infra5_practice1/BEC (May 7, 2015)/Software limit switches/Subsystem/If Action Subsystem ==
  dif : Inport  OutDataType=fixdt(1, 16)  OutScaling=2^0
  Inc : Inport  Port=2  OutDataType=fixdt(1, 16)  OutScaling=2^0
  Action Port : ActionPort  ActionType=then
  PSEA2 : Constant  Value=0  OutDataType=fixdt(1, 16)  OutScaling=2^0
  Switch : Switch  Criteria=u2 > Threshold  Threshold=1  OutDataType=fixdt(1, 16)  OutScaling=2^0
  Out1 : Outport  OutDataType=fixdt(1, 16)  OutScaling=2^0
  wires:
  PSEA2/1 -> Switch/3
  Switch/1 -> Out1/1
  Inc/1 -> Switch/1
  dif/1 -> Switch/2

== system Sim_Forcing_003h_expe_infra5_practice1/BEC (May 7, 2015)/Software limit switches/Subsystem/If Action Subsystem1 ==
  Inc : Inport  OutDataType=fixdt(1, 16)  OutScaling=2^0
  dif : Inport  Port=2  OutDataType=fixdt(1, 16)  OutScaling=2^0
  Action Port : ActionPort  ActionType=else
  PSEA2 : Constant  Value=0  OutDataType=fixdt(1, 16)  OutScaling=2^0
  Switch : Switch  Threshold=1  OutDataType=fixdt(1, 16)  OutScaling=2^0
  Out1 : Outport  OutDataType=fixdt(1, 16)  OutScaling=2^0
  wires:
  dif/1 -> Switch/2
  Inc/1 -> Switch/1
  Switch/1 -> Out1/1
  PSEA2/1 -> Switch/3

== system Sim_Forcing_003h_expe_infra5_practice1/BEC (May 7, 2015)/Software limit switches/Subsystem1/If Action Subsystem ==
  dif : Inport  OutDataType=fixdt(1, 16)  OutScaling=2^0
  Inc : Inport  Port=2  OutDataType=fixdt(1, 16)  OutScaling=2^0
  Action Port : ActionPort  ActionType=then
  PSEA2 : Constant  Value=0  OutDataType=fixdt(1, 16)  OutScaling=2^0
  Switch : Switch  Threshold=1  OutDataType=fixdt(1, 16)  OutScaling=2^0
  Out1 : Outport  OutDataType=fixdt(1, 16)  OutScaling=2^0
  wires:
  dif/1 -> Switch/2
  Inc/1 -> Switch/1
  Switch/1 -> Out1/1
  PSEA2/1 -> Switch/3

== system Sim_Forcing_003h_expe_infra5_practice1/BEC (May 7, 2015)/Software limit switches/Subsystem1/If Action Subsystem1 ==
  Inc : Inport  OutDataType=fixdt(1, 16)  OutScaling=2^0
  dif : Inport  Port=2  OutDataType=fixdt(1, 16)  OutScaling=2^0
  Action Port : ActionPort  ActionType=else
  PSEA2 : Constant  Value=0  OutDataType=fixdt(1, 16)  OutScaling=2^0
  Switch : Switch  Threshold=1  OutDataType=fixdt(1, 16)  OutScaling=2^0
  Out1 : Outport  OutDataType=fixdt(1, 16)  OutScaling=2^0
  wires:
  PSEA2/1 -> Switch/3
  Switch/1 -> Out1/1
  Inc/1 -> Switch/1
  dif/1 -> Switch/2

== system Sim_Forcing_003h_expe_infra5_practice1/BEC (May 7, 2015)/Software limit switches/Subsystem2/If Action Subsystem ==
  dif : Inport  OutDataType=fixdt(1, 16)  OutScaling=2^0
  Inc : Inport  Port=2  OutDataType=fixdt(1, 16)  OutScaling=2^0
  Action Port : ActionPort  ActionType=then
  PSEA2 : Constant  Value=0  OutDataType=fixdt(1, 16)  OutScaling=2^0
  Switch : Switch  Threshold=1  OutDataType=fixdt(1, 16)  OutScaling=2^0
  Out1 : Outport  OutDataType=fixdt(1, 16)  OutScaling=2^0
  wires:
  PSEA2/1 -> Switch/3
  Switch/1 -> Out1/1
  Inc/1 -> Switch/1
  dif/1 -> Switch/2

== system Sim_Forcing_003h_expe_infra5_practice1/BEC (May 7, 2015)/Software limit switches/Subsystem2/If Action Subsystem1 ==
  Inc : Inport  OutDataType=fixdt(1, 16)  OutScaling=2^0
  dif : Inport  Port=2  OutDataType=fixdt(1, 16)  OutScaling=2^0
  Action Port : ActionPort  ActionType=else
  PSEA2 : Constant  Value=0  OutDataType=fixdt(1, 16)  OutScaling=2^0
  Switch : Switch  Threshold=1  OutDataType=fixdt(1, 16)  OutScaling=2^0
  Out1 : Outport  OutDataType=fixdt(1, 16)  OutScaling=2^0
  wires:
  dif/1 -> Switch/2
  Inc/1 -> Switch/1
  Switch/1 -> Out1/1
  PSEA2/1 -> Switch/3

== system Sim_Forcing_003h_expe_infra5_practice1/BEC (May 7, 2015)/Software limit switches/Subsystem3/If Action Subsystem ==
  dif : Inport  OutDataType=fixdt(1, 16)  OutScaling=2^0
  Inc : Inport  Port=2  OutDataType=fixdt(1, 16)  OutScaling=2^0
  Action Port : ActionPort  ActionType=then
  PSEA2 : Constant  Value=0  OutDataType=fixdt(1, 16)  OutScaling=2^0
  Switch : Switch  Threshold=1  OutDataType=fixdt(1, 16)  OutScaling=2^0
  Out1 : Outport  OutDataType=fixdt(1, 16)  OutScaling=2^0
  wires:
  dif/1 -> Switch/2
  Inc/1 -> Switch/1
  Switch/1 -> Out1/1
  PSEA2/1 -> Switch/3

== system Sim_Forcing_003h_expe_infra5_practice1/BEC (May 7, 2015)/Software limit switches/Subsystem3/If Action Subsystem1 ==
  Inc : Inport  OutDataType=fixdt(1, 16)  OutScaling=2^0
  dif : Inport  Port=2  OutDataType=fixdt(1, 16)  OutScaling=2^0
  Action Port : ActionPort  ActionType=else
  PSEA2 : Constant  Value=0  OutDataType=fixdt(1, 16)  OutScaling=2^0
  Switch : Switch  Threshold=1  OutDataType=fixdt(1, 16)  OutScaling=2^0
  Out1 : Outport  OutDataType=fixdt(1, 16)  OutScaling=2^0
  wires:
  PSEA2/1 -> Switch/3
  Switch/1 -> Out1/1
  Inc/1 -> Switch/1
  dif/1 -> Switch/2

== system Sim_Forcing_003h_expe_infra5_practice1/BEC (May 7, 2015)/Software limit switches/Subsystem4/If Action Subsystem ==
  dif : Inport  OutDataType=fixdt(1, 16)  OutScaling=2^0
  Inc : Inport  Port=2  OutDataType=fixdt(1, 16)  OutScaling=2^0
  Action Port : ActionPort  ActionType=then
  PSEA2 : Constant  Value=0  OutDataType=fixdt(1, 16)  OutScaling=2^0
  Switch : Switch  Threshold=1  OutDataType=fixdt(1, 16)  OutScaling=2^0
  Out1 : Outport  OutDataType=fixdt(1, 16)  OutScaling=2^0
  wires:
  PSEA2/1 -> Switch/3
  Switch/1 -> Out1/1
  Inc/1 -> Switch/1
  dif/1 -> Switch/2

== system Sim_Forcing_003h_expe_infra5_practice1/BEC (May 7, 2015)/Software limit switches/Subsystem4/If Action Subsystem1 ==
  Inc : Inport  OutDataType=fixdt(1, 16)  OutScaling=2^0
  dif : Inport  Port=2  OutDataType=fixdt(1, 16)  OutScaling=2^0
  Action Port : ActionPort  ActionType=else
  PSEA2 : Constant  Value=0  OutDataType=fixdt(1, 16)  OutScaling=2^0
  Switch : Switch  Threshold=1  OutDataType=fixdt(1, 16)  OutScaling=2^0
  Out1 : Outport  OutDataType=fixdt(1, 16)  OutScaling=2^0
  wires:
  dif/1 -> Switch/2
  Inc/1 -> Switch/1
  Switch/1 -> Out1/1
  PSEA2/1 -> Switch/3

== system Sim_Forcing_003h_expe_infra5_practice1/BEC (May 7, 2015)/Software limit switches/Subsystem5/If Action Subsystem ==
  dif : Inport  OutDataType=fixdt(1, 16)  OutScaling=2^0
  Inc : Inport  Port=2  OutDataType=fixdt(1, 16)  OutScaling=2^0
  Action Port : ActionPort  ActionType=then
  PSEA2 : Constant  Value=0  OutDataType=fixdt(1, 16)  OutScaling=2^0
  Switch : Switch  Threshold=1  OutDataType=fixdt(1, 16)  OutScaling=2^0
  Out1 : Outport  OutDataType=fixdt(1, 16)  OutScaling=2^0
  wires:
  dif/1 -> Switch/2
  Inc/1 -> Switch/1
  Switch/1 -> Out1/1
  PSEA2/1 -> Switch/3

== system Sim_Forcing_003h_expe_infra5_practice1/BEC (May 7, 2015)/Software limit switches/Subsystem5/If Action Subsystem1 ==
  Inc : Inport  OutDataType=fixdt(1, 16)  OutScaling=2^0
  dif : Inport  Port=2  OutDataType=fixdt(1, 16)  OutScaling=2^0
  Action Port : ActionPort  ActionType=else
  PSEA2 : Constant  Value=0  OutDataType=fixdt(1, 16)  OutScaling=2^0
  Switch : Switch  Threshold=1  OutDataType=fixdt(1, 16)  OutScaling=2^0
  Out1 : Outport  OutDataType=fixdt(1, 16)  OutScaling=2^0
  wires:
  PSEA2/1 -> Switch/3
  Switch/1 -> Out1/1
  Inc/1 -> Switch/1
  dif/1 -> Switch/2

== system Sim_Forcing_003h_expe_infra5_practice1/Breaking_Control 20/07/15/practice_phase1/Rate Control Dynamics Phi/Second-Order Filter, zeta 0.8 ==
  u : Inport
  T : Inport  Port=2  OutDataType=fixdt(1, 16)  OutScaling=2^0
  4*zeta*pi : Gain  Gain=3.2*pi  ParameterDataType=fixdt(1, 16)  ParameterScaling=2^0  OutDataTypeMode=double  OutDataType=fixdt(1, 16)  OutScaling=2^0  OutDataTypeStr=double
  4*zeta*pi/T_transfer /s : DiscreteIntegrator  gainval=1  SampleTime=0.004  OutDataType=fixdt(1, 16)  OutScaling=2^0  ICPrevOutput=DiscIntNeverNeededParam  ICPrevScaledInput=DiscIntNeverNeededParam
  Divide : Product  Inputs=*/  OutDataType=fixdt(1, 16)  OutScaling=2^-10
  Divide1 : Product  Inputs=*/  OutDataType=fixdt(1, 16)  OutScaling=2^-10
  Sum1 : Sum  Inputs=|+-  OutDataType=fixdt(1, 16)  OutScaling=2^0
  Sum2 : Sum  Inputs=-+|  OutDataType=fixdt(1, 16)  OutScaling=2^0
  pi/(zeta*T_transfer)/s : DiscreteIntegrator  gainval=1  SampleTime=0.004  OutDataType=fixdt(1, 16)  OutScaling=2^0  ICPrevOutput=DiscIntNeverNeededParam  ICPrevScaledInput=DiscIntNeverNeededParam
  pi/zeta : Gain  Gain=pi/0.8  ParameterDataType=fixdt(1, 16)  ParameterScaling=2^0  OutDataType=fixdt(1, 16)  OutScaling=2^0
  x : Outport
  wires:
  Divide/1 -> 4*zeta*pi/1
  Divide1/1 -> pi/zeta/1
  pi/zeta/1 -> pi/(zeta*T_transfer)/s/1
  pi/(zeta*T_transfer)/s/1 -> Sum2/1, x/1
  4*zeta*pi/T_transfer /s/1 -> Divide1/1, Sum1/2
  Sum1/1 -> Divide/1
  4*zeta*pi/1 -> 4*zeta*pi/T_transfer /s/1
  T/1 -> [T]
  [T] -> Divide/2
  [T] -> Divide1/2
  Sum2/1 -> Sum1/1
  u/1 -> Sum2/2

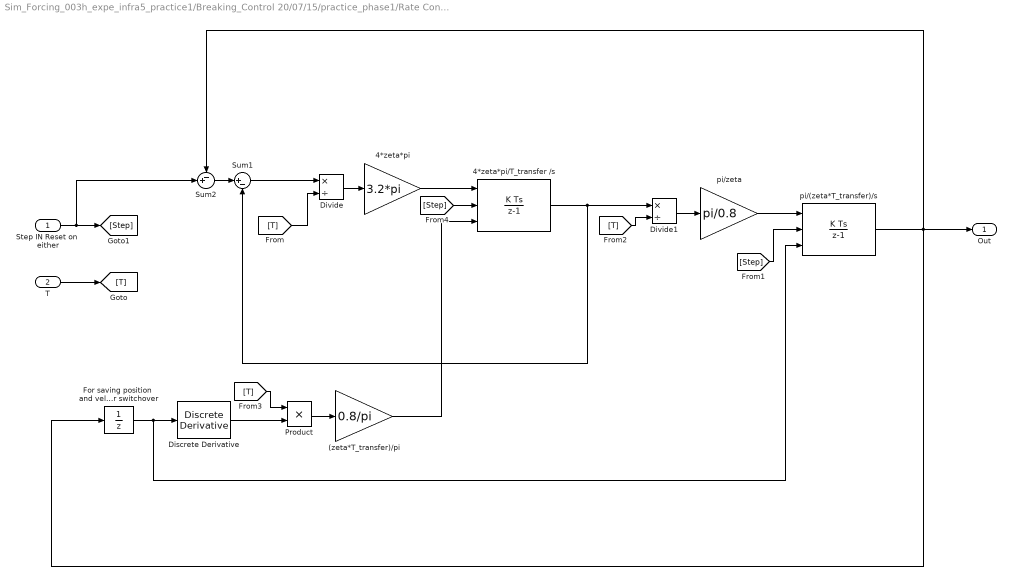
== system Sim_Forcing_003h_expe_infra5_practice1/Breaking_Control 20/07/15/practice_phase1/Rate Control Dynamics Phi/Smooth Displacement Second-Order Filter, zeta 0.8 ==
  Step IN Reset on  either : Inport
  T : Inport  Port=2  OutDataType=fixdt(1, 16)  OutScaling=2^0
  (zeta*T_transfer)/pi : Gain  Gain=0.8/pi  ParameterDataType=fixdt(1, 16)  ParameterScaling=2^0  OutDataType=fixdt(1, 16)  OutScaling=2^0
  4*zeta*pi : Gain  Gain=3.2*pi  ParameterDataType=fixdt(1, 16)  ParameterScaling=2^0  OutDataType=fixdt(1, 16)  OutScaling=2^0
  4*zeta*pi/T_transfer /s : DiscreteIntegrator  gainval=1  ExternalReset=either  InitialConditionSource=external  SampleTime=0.004  OutDataType=fixdt(1, 16)  OutScaling=2^0  ICPrevOutput=DiscIntNeverNeededParam  ICPrevScaledInput=DiscIntNeverNeededParam
  Discrete Derivative : simulink/Discrete/Discrete Derivative  SystemSampleTime=-1  gainval=1.0  ICPrevScaledInput=0.0  OutMin=[]  OutMax=[]  OutDataType=fixdt(1, 16)  OutScaling=2^-10  DoSatur=off
  Divide : Product  Inputs=*/  OutDataType=fixdt(1, 16)  OutScaling=2^-10
  Divide1 : Product  Inputs=*/  OutDataType=fixdt(1, 16)  OutScaling=2^-10
  For saving position  and velocity until after switchover : UnitDelay  SampleTime=-1
  Product : Product  OutDataType=fixdt(1, 16)  OutScaling=2^0  RndMeth=Zero
  Sum1 : Sum  Inputs=|+-  OutDataType=fixdt(1, 16)  OutScaling=2^0
  Sum2 : Sum  Inputs=-+|  OutDataType=fixdt(1, 16)  OutScaling=2^0
  pi/(zeta*T_transfer)/s : DiscreteIntegrator  gainval=1  ExternalReset=either  InitialConditionSource=external  SampleTime=0.004  OutDataType=fixdt(1, 16)  OutScaling=2^0  ICPrevOutput=DiscIntNeverNeededParam  ICPrevScaledInput=DiscIntNeverNeededParam
  pi/zeta : Gain  Gain=pi/0.8  ParameterDataType=fixdt(1, 16)  ParameterScaling=2^0  OutDataType=fixdt(1, 16)  OutScaling=2^0
  Out : Outport
  wires:
  Discrete Derivative/1 -> Product/2
  Product/1 -> (zeta*T_transfer)/pi/1
  Divide/1 -> 4*zeta*pi/1
  Divide1/1 -> pi/zeta/1
  pi/zeta/1 -> pi/(zeta*T_transfer)/s/1
  pi/(zeta*T_transfer)/s/1 -> Sum2/1, Out/1, For saving position  and velocity until after switchover/1
  4*zeta*pi/T_transfer /s/1 -> Divide1/1, Sum1/2
  Sum1/1 -> Divide/1
  4*zeta*pi/1 -> 4*zeta*pi/T_transfer /s/1
  T/1 -> [T]
  Step IN Reset on  either/1 -> [Step], Sum2/2
  [Step] -> 4*zeta*pi/T_transfer /s/2
  [Step] -> pi/(zeta*T_transfer)/s/2
  [T] -> Divide/2
  For saving position  and velocity until after switchover/1 -> Discrete Derivative/1, pi/(zeta*T_transfer)/s/3
  [T] -> Product/1
  (zeta*T_transfer)/pi/1 -> 4*zeta*pi/T_transfer /s/3
  [T] -> Divide1/2
  Sum2/1 -> Sum1/1

== system Sim_Forcing_003h_expe_infra5_practice1/Breaking_Control 20/07/15/practice_phase1/Rate Control Dynamics Psi2/Arm-filter ==
  u : Inport
  2*zeta*om : Inport  Port=2
  om^2 : Inport  Port=3
  reset : Inport  Port=4
  Discrete-Time Integrator : DiscreteIntegrator  ExternalReset=either  SampleTime=0.004  ICPrevOutput=DiscIntNeverNeededParam  ICPrevScaledInput=DiscIntNeverNeededParam
  Discrete-Time Integrator1 : DiscreteIntegrator  ExternalReset=either  SampleTime=0.004  ICPrevOutput=DiscIntNeverNeededParam  ICPrevScaledInput=DiscIntNeverNeededParam
  Product{,1..3} (4 alike) : Product  RndMeth=Zero
  Sum4 : Sum  Inputs=+|-|-
  Sum5 : Sum  Inputs=++|
  x : Outport
  wires:
  om^2/1 -> Product1/1, Product/1
  u/1 -> Product3/2, Product/2
  Product2/1 -> Sum4/3
  Product1/1 -> Sum4/2
  Product/1 -> Sum4/1
  2*zeta*om/1 -> Product3/1, Product2/1
  Sum5/1 -> Product2/2, Discrete-Time Integrator/1
  Discrete-Time Integrator/1 -> x/1, Product1/2
  Product3/1 -> Sum5/1
  Sum4/1 -> Discrete-Time Integrator1/1
  Discrete-Time Integrator1/1 -> Sum5/2
  reset/1 -> Discrete-Time Integrator1/2, Discrete-Time Integrator/2

== system Sim_Forcing_003h_expe_infra5_practice1/Breaking_Control 20/07/15/practice_phase1/Rate Control Dynamics Psi2/Cabin-Filter ==
  u : Inport
  2*zeta*om : Inport  Port=2
  om^2 : Inport  Port=3
  reset : Inport  Port=4
  Discrete-Time Integrator : DiscreteIntegrator  ExternalReset=either  SampleTime=0.004  ICPrevOutput=DiscIntNeverNeededParam  ICPrevScaledInput=DiscIntNeverNeededParam
  Discrete-Time Integrator1 : DiscreteIntegrator  ExternalReset=either  SampleTime=0.004  ICPrevOutput=DiscIntNeverNeededParam  ICPrevScaledInput=DiscIntNeverNeededParam
  Product1 : Product  RndMeth=Zero
  Product2 : Product  RndMeth=Zero
  Sum4 : Sum  Inputs=+|-|-
  x_2dot : Outport
  x_dot : Outport  Port=2
  wires:
  om^2/1 -> Product1/1
  Product2/1 -> Sum4/3
  Product1/1 -> Sum4/2
  2*zeta*om/1 -> Product2/1
  Discrete-Time Integrator1/1 -> Product2/2, x_dot/1, Discrete-Time Integrator/1
  Discrete-Time Integrator/1 -> Product1/2
  Sum4/1 -> x_2dot/1, Discrete-Time Integrator1/1
  u/1 -> Sum4/1
  reset/1 -> Discrete-Time Integrator1/2, Discrete-Time Integrator/2

== system Sim_Forcing_003h_expe_infra5_practice1/Breaking_Control 20/07/15/practice_phase1/Rate Control Dynamics Psi2/Second-Order Filter, zeta 0.8 ==
  u : Inport
  T : Inport  Port=2  OutDataType=fixdt(1, 16)  OutScaling=2^0
  reset : Inport  Port=3  OutDataType=fixdt(1, 16)  OutScaling=2^0
  4*zeta*pi : Gain  Gain=3.2*pi  ParameterDataType=fixdt(1, 16)  ParameterScaling=2^0  OutDataTypeMode=double  OutDataType=fixdt(1, 16)  OutScaling=2^0  OutDataTypeStr=double
  4*zeta*pi/T_transfer /s : DiscreteIntegrator  gainval=1  ExternalReset=either  SampleTime=0.004  OutDataType=fixdt(1, 16)  OutScaling=2^0  ICPrevOutput=DiscIntNeverNeededParam  ICPrevScaledInput=DiscIntNeverNeededParam
  Divide : Product  Inputs=*/  OutDataType=fixdt(1, 16)  OutScaling=2^-10
  Divide1 : Product  Inputs=*/  OutDataType=fixdt(1, 16)  OutScaling=2^-10
  Sum1 : Sum  Inputs=|+-  OutDataType=fixdt(1, 16)  OutScaling=2^0
  Sum2 : Sum  Inputs=-+|  OutDataType=fixdt(1, 16)  OutScaling=2^0
  pi/(zeta*T_transfer)/s : DiscreteIntegrator  gainval=1  ExternalReset=either  SampleTime=0.004  OutDataType=fixdt(1, 16)  OutScaling=2^0  ICPrevOutput=DiscIntNeverNeededParam  ICPrevScaledInput=DiscIntNeverNeededParam
  pi/zeta : Gain  Gain=pi/0.8  ParameterDataType=fixdt(1, 16)  ParameterScaling=2^0  OutDataType=fixdt(1, 16)  OutScaling=2^0
  x : Outport
  wires:
  Divide/1 -> 4*zeta*pi/1
  Divide1/1 -> pi/zeta/1
  pi/zeta/1 -> pi/(zeta*T_transfer)/s/1
  pi/(zeta*T_transfer)/s/1 -> Sum2/1, x/1
  4*zeta*pi/T_transfer /s/1 -> Divide1/1, Sum1/2
  Sum1/1 -> Divide/1
  4*zeta*pi/1 -> 4*zeta*pi/T_transfer /s/1
  T/1 -> [T]
  [T] -> Divide/2
  [T] -> Divide1/2
  Sum2/1 -> Sum1/1
  u/1 -> Sum2/2
  reset/1 -> 4*zeta*pi/T_transfer /s/2, pi/(zeta*T_transfer)/s/2
